simulink model "check_Engine"  (R2018b)
settings: configuration reference "Physics" (kept outside this file)
model workspace (MAT data in the model file):
  veh_param = Simulink.Parameter
  veh_param.Value.cLiftF = 0
  veh_param.Value.cLiftR = 0
  veh_param.Value.CoGx_m = 0
  veh_param.Value.CoGy_m = 0
  veh_param.Value.CoGz_m = 0
  veh_param.Value.cDrag = 0
  veh_param.Value.Aref_m2 = 0
  veh_param.Value.Gearratio = 0
  veh_param.Value.Wheelbase_m = 0
  veh_param.Value.PacLatF = [0 0 0 0 0]
  veh_param.Value.PacLongF = [0 0 0 0 0]
  veh_param.Value.PacLatR = [0 0 0 0 0]
  veh_param.Value.PacLongR = [0 0 0 0 0]
  veh_param.Value.cRollFriction_Npmps = 0
  veh_param.Value.MaxRollFriction_N = 0
  veh_param.Value.T_YawRate_s = 0
  veh_param.Value.T_LatVel_s = 0
  veh_param.Value.TrackWidthF_m = 0
  veh_param.Value.TrackWidthR_m = 0
  veh_param.Value.TireRadiusF_m = 0
  veh_param.Value.TireRadiusR_m = 0
  veh_param.Value.VehicleInertia_kgm2 = 0
  veh_param.Value.WheelInertiaF_kgm2 = 0
  veh_param.Value.WheelInertiaR_kgm2 = 0
  veh_param.Value.VehicleMass_kg = 0
  veh_param.Value.switchModelBlend_mps = 0
  veh_param.Value.PTLimitLowVel_N = 0
  veh_param.Value.switchModelVel_mps = 0
  veh_param.Value.T_Tire_s = 0
  veh_param.DataType = 'struct'
  veh_param.Dimensions = [1 1]
  x0_positionstates = Simulink.Parameter
  x0_positionstates.Value = [0 0 0]
  x0_positionstates.DataType = 'auto'
  x0_positionstates.Dimensions = [1 3]
undefined symbols (not defined in the file): POWTR__DIFFERENTIAL__c_diff_efficiency, POWTR__DIFFERENTIAL__c_diff_ratio, POWTR__DIFFERENTIAL__f_diff_efficiency, POWTR__DIFFERENTIAL__f_diff_ratio, POWTR__DIFFERENTIAL__r_diff_efficiency, POWTR__DIFFERENTIAL__r_diff_ratio, POWTR__ENGINE__n_idle_rpm, POWTR__ENGINE__n_lb_rpm__1, POWTR__ENGINE__n_lb_rpm__2, POWTR__ENGINE__n_lb_rpm__3, POWTR__ENGINE__n_lb_rpm__4, POWTR__ENGINE__n_lb_rpm__5, POWTR__ENGINE__n_lb_rpm__6, POWTR__ENGINE__n_lb_rpm__7, POWTR__ENGINE__n_limit_rpm, POWTR__LAYOUT__p_torque_rear, POWTR__MODE__activate_ThrottleInterface, POWTR__TRANSMISSION__gear__1, POWTR__TRANSMISSION__gear__2, POWTR__TRANSMISSION__gear__3, POWTR__TRANSMISSION__gear__4, POWTR__TRANSMISSION__gear__5, POWTR__TRANSMISSION__gear__6, POWTR__TRANSMISSION__gear__7, POWTR__TRANSMISSION__gear_efficiency__1, POWTR__TRANSMISSION__gear_efficiency__2, POWTR__TRANSMISSION__gear_efficiency__3, POWTR__TRANSMISSION__gear_efficiency__4, POWTR__TRANSMISSION__gear_efficiency__5, POWTR__TRANSMISSION__gear_efficiency__6, POWTR__TRANSMISSION__gear_efficiency__7, POWTR__TRANSMISSION__gear_ratio__1, POWTR__TRANSMISSION__gear_ratio__2, POWTR__TRANSMISSION__gear_ratio__3, POWTR__TRANSMISSION__gear_ratio__4, POWTR__TRANSMISSION__gear_ratio__5, POWTR__TRANSMISSION__gear_ratio__6, POWTR__TRANSMISSION__gear_ratio__7, tireFL__MFSIMPLE__r_tire_m, tireFR__MFSIMPLE__r_tire_m, tireRL__MFSIMPLE__r_tire_m, tireRR__MFSIMPLE__r_tire_m
libraries: simulink x3
settings Model: DataDictionary=vehicleparameters_vehdynsim.sldd  OrderedModelArguments=off  Creator=wischnewski  LastModifiedBy=ga25xiw

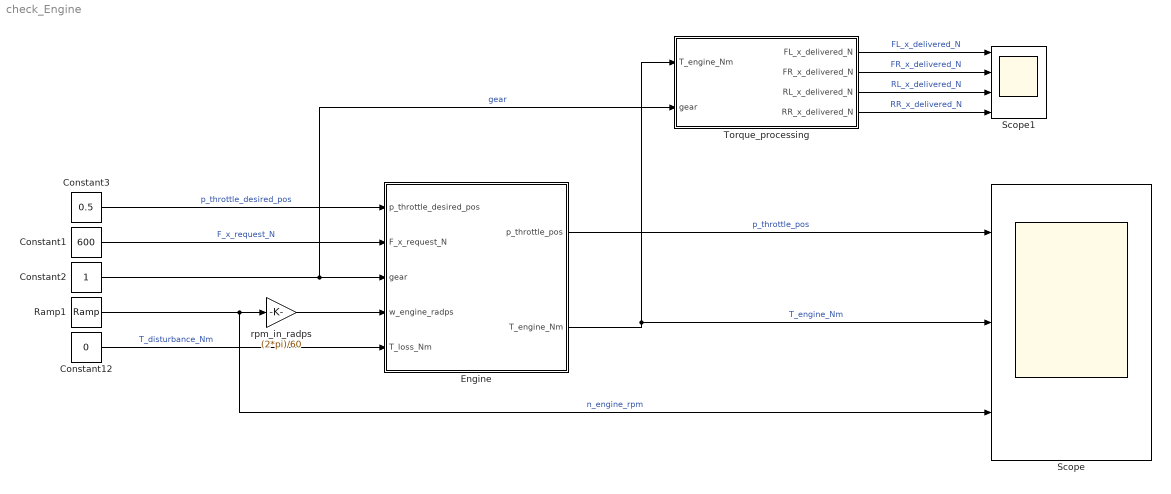
== system check_Engine ==
  Constant1 : Constant  Value=600
  Constant12 : Constant  Value=0
  Constant2 : Constant
  Constant3 : Constant  Value=0.5
  Engine : Subsystem
  Ramp1 : simulink/Sources/Ramp  slope=500  start=0  InitialOutput=2000
  Scope : Scope  NumInputPorts=3
  Scope1 : Scope  NumInputPorts=4
  Torque_processing : Subsystem
  rpm_in_radps : Gain  Gain=(2*pi)/60
  wires:
  Ramp1/1 -> Scope/3, rpm_in_radps/1  "n_engine_rpm"
  Engine/1(p_throttle_pos) -> Scope/1  "p_throttle_pos"
  Torque_processing/1(FL_x_delivered_N) -> Scope1/1  "FL_x_delivered_N"
  Torque_processing/2(FR_x_delivered_N) -> Scope1/2  "FR_x_delivered_N"
  Torque_processing/3(RL_x_delivered_N) -> Scope1/3  "RL_x_delivered_N"
  Torque_processing/4(RR_x_delivered_N) -> Scope1/4  "RR_x_delivered_N"
  Engine/2(T_engine_Nm) -> Torque_processing/1(T_engine_Nm), Scope/2  "T_engine_Nm"
  Constant12/1 -> Engine/5(T_loss_Nm)  "T_disturbance_Nm"
  rpm_in_radps/1 -> Engine/4(w_engine_radps)
  Constant2/1 -> Engine/3(gear), Torque_processing/2(gear)  "gear"
  Constant1/1 -> Engine/2(F_x_request_N)  "F_x_request_N"
  Constant3/1 -> Engine/1(p_throttle_desired_pos)  "p_throttle_desired_pos"

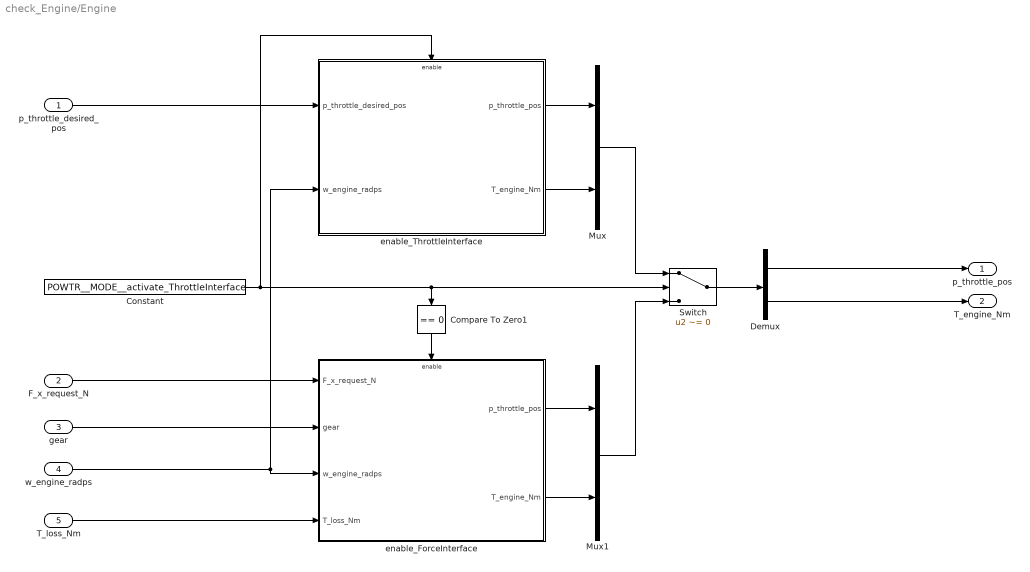
== system check_Engine/Engine ==
  p_throttle_desired_pos : Inport
  F_x_request_N : Inport  Port=2
  gear : Inport  Port=3
  w_engine_radps : Inport  Port=4
  T_loss_Nm : Inport  Port=5
  Compare To Zero1 : simulink/Logic and Bit Operations/Compare To Zero  relop===  OutDataTypeStr=uint8
  Constant : Constant  Value=POWTR__MODE__activate_ThrottleInterface
  Demux : Demux  Outputs=2
  Mux : Mux  Inputs=2
  Mux1 : Mux  Inputs=2
  Switch : Switch  Criteria=u2 ~= 0
  enable_ForceInterface : Subsystem
  enable_ThrottleInterface : Subsystem
  p_throttle_pos : Outport
  T_engine_Nm : Outport  Port=2
  wires:
  Switch/1 -> Demux/1
  Mux1/1 -> Switch/3
  Compare To Zero1/1 -> enable_ForceInterface/Enable
  T_loss_Nm/1 -> enable_ForceInterface/4(T_loss_Nm)
  gear/1 -> enable_ForceInterface/2(gear)
  w_engine_radps/1 -> enable_ForceInterface/3(w_engine_radps), enable_ThrottleInterface/2(w_engine_radps)
  enable_ForceInterface/2(T_engine_Nm) -> Mux1/2
  Constant/1 -> Switch/2, Compare To Zero1/1, enable_ThrottleInterface/Enable
  enable_ForceInterface/1(p_throttle_pos) -> Mux1/1
  F_x_request_N/1 -> enable_ForceInterface/1(F_x_request_N)
  p_throttle_desired_pos/1 -> enable_ThrottleInterface/1(p_throttle_desired_pos)
  enable_ThrottleInterface/2(T_engine_Nm) -> Mux/2
  Mux/1 -> Switch/1
  enable_ThrottleInterface/1(p_throttle_pos) -> Mux/1
  Demux/2 -> T_engine_Nm/1
  Demux/1 -> p_throttle_pos/1

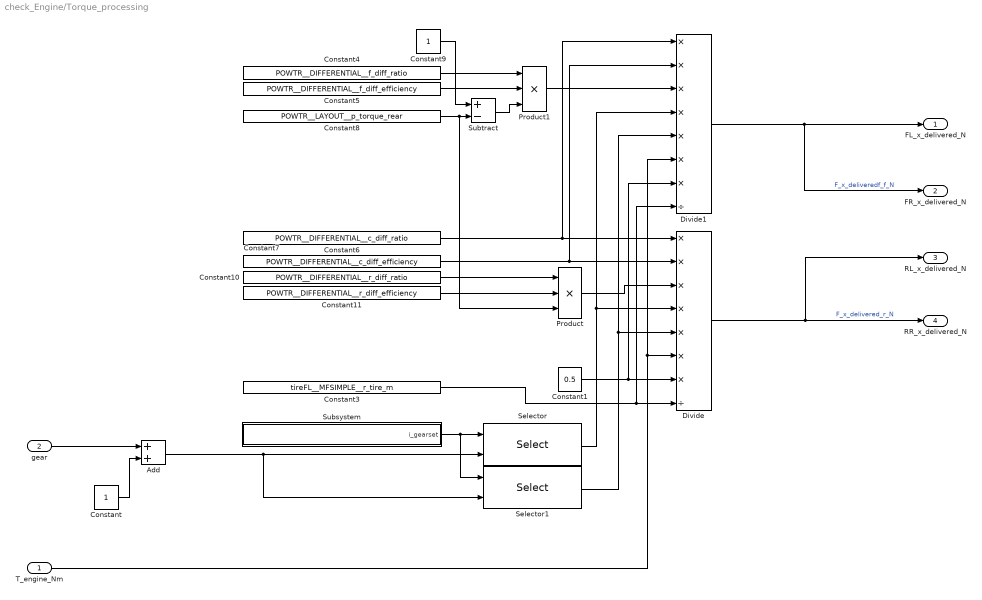
== system check_Engine/Torque_processing ==
  T_engine_Nm : Inport
  gear : Inport  Port=2
  Add : Sum
  Constant : Constant
  Constant1 : Constant  Value=0.5
  Constant10 : Constant  Value=POWTR__DIFFERENTIAL__r_diff_ratio
  Constant11 : Constant  Value=POWTR__DIFFERENTIAL__r_diff_efficiency  VectorParams1D=off
  Constant3 : Constant  Value=tireFL__MFSIMPLE__r_tire_m  VectorParams1D=off
  Constant4 : Constant  Value=POWTR__DIFFERENTIAL__f_diff_ratio
  Constant5 : Constant  Value=POWTR__DIFFERENTIAL__f_diff_efficiency  VectorParams1D=off
  Constant6 : Constant  Value=POWTR__DIFFERENTIAL__c_diff_ratio
  Constant7 : Constant  Value=POWTR__DIFFERENTIAL__c_diff_efficiency
  Constant8 : Constant  Value=POWTR__LAYOUT__p_torque_rear  VectorParams1D=off
  Constant9 : Constant
  Divide : Product  Inputs=*******/
  Divide1 : Product  Inputs=*******/
  Product : Product  Inputs=3
  Product1 : Product  Inputs=3
  Selector : Selector  NumberOfDimensions=2  InputPortWidth=3  IndexOptions=Index vector (dialog),Index vector (port)  Indices=2,1  OutputSizes=1,1
  Selector1 : Selector  NumberOfDimensions=2  InputPortWidth=3  IndexOptions=Index vector (dialog),Index vector (port)  Indices=4,1  OutputSizes=1,1
  Subsystem : Subsystem
  Subtract : Sum  Inputs=+-
  FL_x_delivered_N : Outport
  FR_x_delivered_N : Outport  Port=2
  RL_x_delivered_N : Outport  Port=3
  RR_x_delivered_N : Outport  Port=4
  wires:
  Constant10/1 -> Product/1
  Constant/1 -> Add/2
  Constant8/1 -> Product/3, Subtract/2
  Subsystem/1(i_gearset) -> Selector/1, Selector1/1
  Add/1 -> Selector1/2, Selector/2
  Constant7/1 -> Divide/2, Divide1/2
  Constant9/1 -> Subtract/1
  Constant5/1 -> Product1/2
  Constant6/1 -> Divide/1, Divide1/1
  Subtract/1 -> Product1/3
  Constant4/1 -> Product1/1
  Constant11/1 -> Product/2
  Selector/1 -> Divide/4, Divide1/4
  Selector1/1 -> Divide/5, Divide1/5
  gear/1 -> Add/1
  Product/1 -> Divide/3
  T_engine_Nm/1 -> Divide/6, Divide1/6
  Constant3/1 -> Divide/8, Divide1/8
  Constant1/1 -> Divide/7, Divide1/7
  Product1/1 -> Divide1/3
  Divide/1 -> RL_x_delivered_N/1, RR_x_delivered_N/1  "F_x_delivered_r_N"
  Divide1/1 -> FR_x_delivered_N/1, FL_x_delivered_N/1  "F_x_deliveredf_f_N"

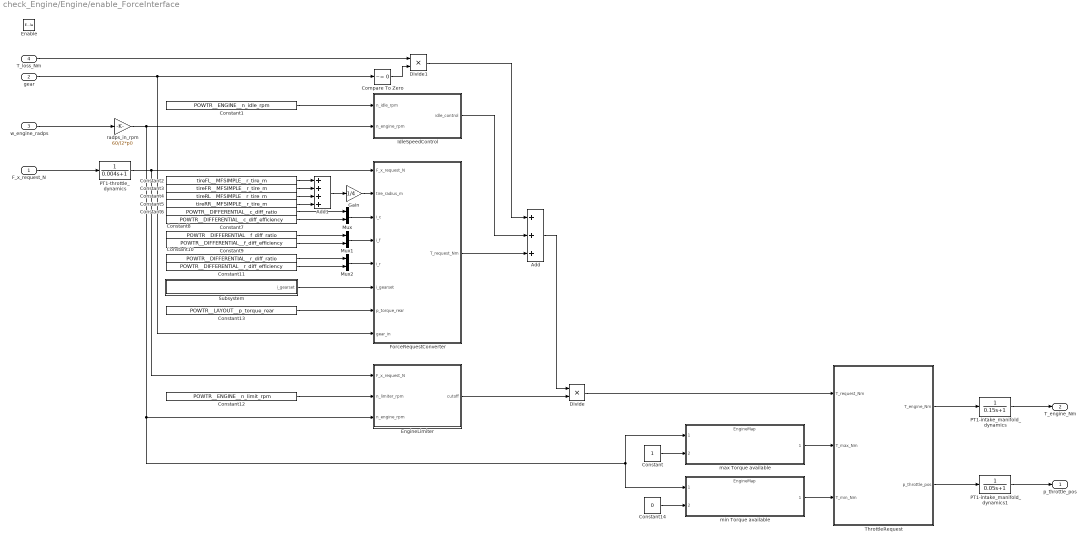
== system check_Engine/Engine/enable_ForceInterface ==
  F_x_request_N : Inport
  gear : Inport  Port=2
  w_engine_radps : Inport  Port=3
  T_loss_Nm : Inport  Port=4
  Enable : EnablePort
  Add : Sum  Inputs=+++
  Add1 : Sum  Inputs=++++
  Compare To Zero : simulink/Logic and Bit Operations/Compare To Zero  relop=~=  OutDataTypeStr=boolean
  Constant : Constant
  Constant1 : Constant  Value=POWTR__ENGINE__n_idle_rpm
  Constant10 : Constant  Value=POWTR__DIFFERENTIAL__r_diff_ratio
  Constant11 : Constant  Value=POWTR__DIFFERENTIAL__r_diff_efficiency
  Constant12 : Constant  Value=POWTR__ENGINE__n_limit_rpm
  Constant13 : Constant  Value=POWTR__LAYOUT__p_torque_rear
  Constant14 : Constant  Value=0
  Constant2 : Constant  Value=tireFL__MFSIMPLE__r_tire_m
  Constant3 : Constant  Value=tireFR__MFSIMPLE__r_tire_m
  Constant4 : Constant  Value=tireRL__MFSIMPLE__r_tire_m
  Constant5 : Constant  Value=tireRR__MFSIMPLE__r_tire_m
  Constant6 : Constant  Value=POWTR__DIFFERENTIAL__c_diff_ratio
  Constant7 : Constant  Value=POWTR__DIFFERENTIAL__c_diff_efficiency
  Constant8 : Constant  Value=POWTR__DIFFERENTIAL__f_diff_ratio
  Constant9 : Constant  Value=POWTR__DIFFERENTIAL__f_diff_efficiency
  Divide : Product  Inputs=**
  Divide1 : Product  Inputs=**
  EngineLimiter : MATLAB Function  TreatAsAtomicUnit=on
  ForceRequestConverter : MATLAB Function  TreatAsAtomicUnit=on
  Gain : Gain  Gain=1/4
  IdleSpeedControl : MATLAB Function  TreatAsAtomicUnit=on
  Mux : Mux  Inputs=2
  Mux1 : Mux  Inputs=2
  Mux2 : Mux  Inputs=2
  PT1-intake_manifold_dynamics : TransferFcn  Denominator=[0.15 1]
  PT1-intake_manifold_dynamics1 : TransferFcn  Denominator=[0.05 1]
  PT1-throttle_dynamics : TransferFcn  Denominator=[0.004 1]
  Subsystem : Subsystem
  ThrottleRequest : MATLAB Function  TreatAsAtomicUnit=on
  max Torque available : ModelReference  ModelNameDialog=EngineMap.slx  SimulationMode=Normal  ModelReferenceVersion=1.393
  min Torque available : ModelReference  ModelNameDialog=EngineMap.slx  SimulationMode=Normal  ModelReferenceVersion=1.393
  radps_in_rpm : Gain  Gain=60/(2*pi)
  p_throttle_pos : Outport
  T_engine_Nm : Outport  Port=2
  wires:
  Constant8/1 -> Mux1/1
  gear/1 -> Compare To Zero/1, ForceRequestConverter/8(gear_in)
  PT1-throttle_dynamics/1 -> ForceRequestConverter/1(F_x_request_N), EngineLimiter/1(F_x_request_N)
  Constant5/1 -> Add1/4
  Constant13/1 -> ForceRequestConverter/7(p_torque_rear)
  Constant7/1 -> Mux/2
  Compare To Zero/1 -> Divide1/2
  T_loss_Nm/1 -> Divide1/1
  EngineLimiter/1(cutoff) -> Divide/2
  Constant3/1 -> Add1/2
  Constant12/1 -> EngineLimiter/2(n_limiter_rpm)
  ForceRequestConverter/1(T_request_Nm) -> Add/3
  Add1/1 -> Gain/1
  IdleSpeedControl/1(idle_control) -> Add/2
  PT1-intake_manifold_dynamics1/1 -> p_throttle_pos/1
  Constant4/1 -> Add1/3
  Mux2/1 -> ForceRequestConverter/5(i_r)
  Divide1/1 -> Add/1
  Constant11/1 -> Mux2/2
  ThrottleRequest/1(T_engine_Nm) -> PT1-intake_manifold_dynamics/1
  Constant10/1 -> Mux2/1
  Mux/1 -> ForceRequestConverter/3(i_c)
  Constant2/1 -> Add1/1
  ThrottleRequest/2(p_throttle_pos) -> PT1-intake_manifold_dynamics1/1
  Mux1/1 -> ForceRequestConverter/4(i_f)
  PT1-intake_manifold_dynamics/1 -> T_engine_Nm/1
  F_x_request_N/1 -> PT1-throttle_dynamics/1
  Add/1 -> Divide/1
  Subsystem/1(i_gearset) -> ForceRequestConverter/6(i_gearset)
  Constant9/1 -> Mux1/2
  w_engine_radps/1 -> radps_in_rpm/1
  Constant1/1 -> IdleSpeedControl/1(n_idle_rpm)
  Gain/1 -> ForceRequestConverter/2(tire_radius_m)
  Constant6/1 -> Mux/1
  Constant14/1 -> min Torque available/2
  radps_in_rpm/1 -> IdleSpeedControl/2(n_engine_rpm), EngineLimiter/3(n_engine_rpm), min Torque available/1, max Torque available/1
  min Torque available/1 -> ThrottleRequest/3(T_min_Nm)
  Divide/1 -> ThrottleRequest/1(T_request_Nm)
  max Torque available/1 -> ThrottleRequest/2(T_max_Nm)
  Constant/1 -> max Torque available/2

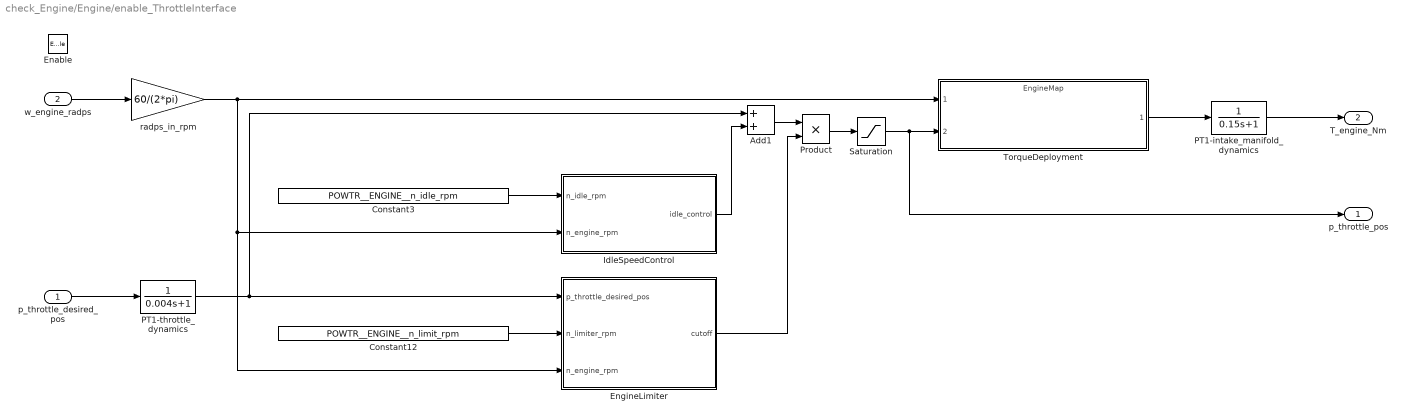
== system check_Engine/Engine/enable_ThrottleInterface ==
  p_throttle_desired_pos : Inport
  w_engine_radps : Inport  Port=2
  Enable : EnablePort
  Add1 : Sum
  Constant12 : Constant  Value=POWTR__ENGINE__n_limit_rpm
  Constant3 : Constant  Value=POWTR__ENGINE__n_idle_rpm
  EngineLimiter : MATLAB Function  TreatAsAtomicUnit=on
  IdleSpeedControl : MATLAB Function  TreatAsAtomicUnit=on
  PT1-intake_manifold_dynamics : TransferFcn  Denominator=[0.15 1]
  PT1-throttle_dynamics : TransferFcn  Denominator=[0.004 1]
  Product : Product
  Saturation : Saturate  UpperLimit=1  LowerLimit=0
  TorqueDeployment : ModelReference  ModelNameDialog=EngineMap.slx  SimulationMode=Normal  ModelReferenceVersion=1.393
  radps_in_rpm : Gain  Gain=60/(2*pi)
  p_throttle_pos : Outport
  T_engine_Nm : Outport  Port=2
  wires:
  Constant12/1 -> EngineLimiter/2(n_limiter_rpm)
  Product/1 -> Saturation/1
  Add1/1 -> Product/1
  EngineLimiter/1(cutoff) -> Product/2
  IdleSpeedControl/1(idle_control) -> Add1/2
  w_engine_radps/1 -> radps_in_rpm/1
  p_throttle_desired_pos/1 -> PT1-throttle_dynamics/1
  Saturation/1 -> TorqueDeployment/2, p_throttle_pos/1
  PT1-intake_manifold_dynamics/1 -> T_engine_Nm/1
  TorqueDeployment/1 -> PT1-intake_manifold_dynamics/1
  radps_in_rpm/1 -> EngineLimiter/3(n_engine_rpm), IdleSpeedControl/2(n_engine_rpm), TorqueDeployment/1
  PT1-throttle_dynamics/1 -> Add1/1, EngineLimiter/1(p_throttle_desired_pos)
  Constant3/1 -> IdleSpeedControl/1(n_idle_rpm)

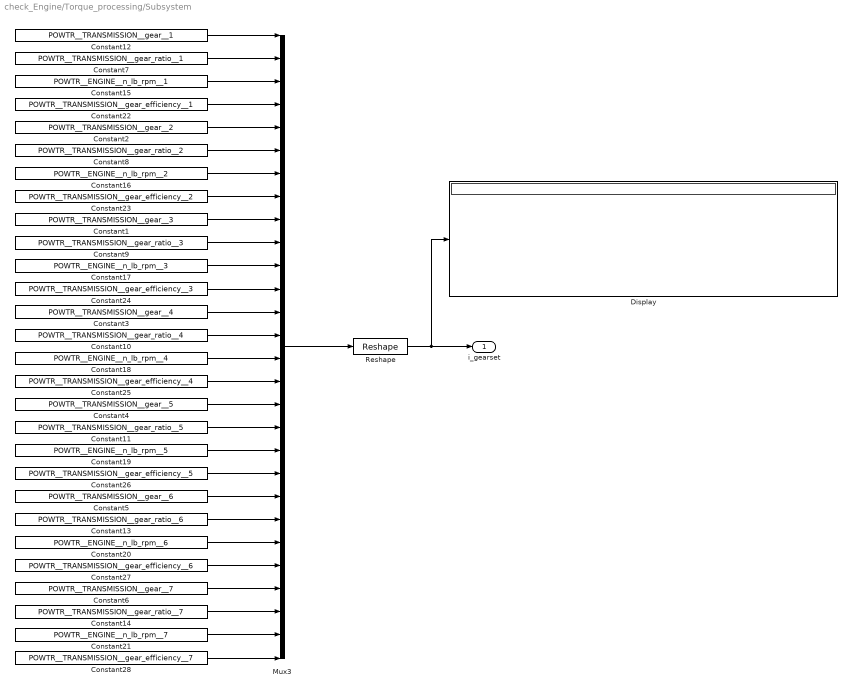
== system check_Engine/Torque_processing/Subsystem ==
  Constant1 : Constant  Value=POWTR__TRANSMISSION__gear__3
  Constant10 : Constant  Value=POWTR__TRANSMISSION__gear_ratio__4
  Constant11 : Constant  Value=POWTR__TRANSMISSION__gear_ratio__5
  Constant12 : Constant  Value=POWTR__TRANSMISSION__gear__1
  Constant13 : Constant  Value=POWTR__TRANSMISSION__gear_ratio__6
  Constant14 : Constant  Value=POWTR__TRANSMISSION__gear_ratio__7
  Constant15 : Constant  Value=POWTR__ENGINE__n_lb_rpm__1
  Constant16 : Constant  Value=POWTR__ENGINE__n_lb_rpm__2
  Constant17 : Constant  Value=POWTR__ENGINE__n_lb_rpm__3
  Constant18 : Constant  Value=POWTR__ENGINE__n_lb_rpm__4
  Constant19 : Constant  Value=POWTR__ENGINE__n_lb_rpm__5
  Constant2 : Constant  Value=POWTR__TRANSMISSION__gear__2
  Constant20 : Constant  Value=POWTR__ENGINE__n_lb_rpm__6
  Constant21 : Constant  Value=POWTR__ENGINE__n_lb_rpm__7
  Constant22 : Constant  Value=POWTR__TRANSMISSION__gear_efficiency__1
  Constant23 : Constant  Value=POWTR__TRANSMISSION__gear_efficiency__2
  Constant24 : Constant  Value=POWTR__TRANSMISSION__gear_efficiency__3
  Constant25 : Constant  Value=POWTR__TRANSMISSION__gear_efficiency__4
  Constant26 : Constant  Value=POWTR__TRANSMISSION__gear_efficiency__5
  Constant27 : Constant  Value=POWTR__TRANSMISSION__gear_efficiency__6
  Constant28 : Constant  Value=POWTR__TRANSMISSION__gear_efficiency__7
  Constant3 : Constant  Value=POWTR__TRANSMISSION__gear__4
  Constant4 : Constant  Value=POWTR__TRANSMISSION__gear__5
  Constant5 : Constant  Value=POWTR__TRANSMISSION__gear__6
  Constant6 : Constant  Value=POWTR__TRANSMISSION__gear__7
  Constant7 : Constant  Value=POWTR__TRANSMISSION__gear_ratio__1
  Constant8 : Constant  Value=POWTR__TRANSMISSION__gear_ratio__2
  Constant9 : Constant  Value=POWTR__TRANSMISSION__gear_ratio__3
  Display : Display
  Mux3 : Mux  Inputs=28
  Reshape : Reshape  OutputDimensionality=Customize  OutputDimensions=[4,7]
  i_gearset : Outport
  wires:
  Mux3/1 -> Reshape/1
  Constant12/1 -> Mux3/1
  Reshape/1 -> i_gearset/1, Display/1
  Constant2/1 -> Mux3/5
  Constant1/1 -> Mux3/9
  Constant3/1 -> Mux3/13
  Constant4/1 -> Mux3/17
  Constant5/1 -> Mux3/21
  Constant6/1 -> Mux3/25
  Constant7/1 -> Mux3/2
  Constant8/1 -> Mux3/6
  Constant9/1 -> Mux3/10
  Constant10/1 -> Mux3/14
  Constant11/1 -> Mux3/18
  Constant13/1 -> Mux3/22
  Constant14/1 -> Mux3/26
  Constant15/1 -> Mux3/3
  Constant16/1 -> Mux3/7
  Constant17/1 -> Mux3/11
  Constant18/1 -> Mux3/15
  Constant19/1 -> Mux3/19
  Constant20/1 -> Mux3/23
  Constant21/1 -> Mux3/27
  Constant22/1 -> Mux3/4
  Constant23/1 -> Mux3/8
  Constant24/1 -> Mux3/12
  Constant25/1 -> Mux3/16
  Constant26/1 -> Mux3/20
  Constant27/1 -> Mux3/24
  Constant28/1 -> Mux3/28

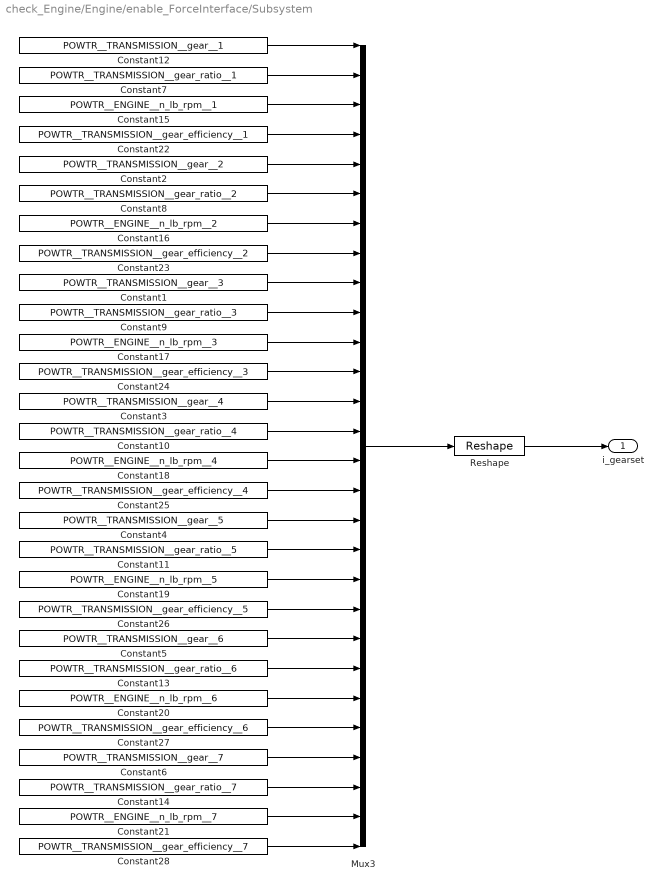
== system check_Engine/Engine/enable_ForceInterface/Subsystem ==
  Constant1 : Constant  Value=POWTR__TRANSMISSION__gear__3
  Constant10 : Constant  Value=POWTR__TRANSMISSION__gear_ratio__4
  Constant11 : Constant  Value=POWTR__TRANSMISSION__gear_ratio__5
  Constant12 : Constant  Value=POWTR__TRANSMISSION__gear__1
  Constant13 : Constant  Value=POWTR__TRANSMISSION__gear_ratio__6
  Constant14 : Constant  Value=POWTR__TRANSMISSION__gear_ratio__7
  Constant15 : Constant  Value=POWTR__ENGINE__n_lb_rpm__1
  Constant16 : Constant  Value=POWTR__ENGINE__n_lb_rpm__2
  Constant17 : Constant  Value=POWTR__ENGINE__n_lb_rpm__3
  Constant18 : Constant  Value=POWTR__ENGINE__n_lb_rpm__4
  Constant19 : Constant  Value=POWTR__ENGINE__n_lb_rpm__5
  Constant2 : Constant  Value=POWTR__TRANSMISSION__gear__2
  Constant20 : Constant  Value=POWTR__ENGINE__n_lb_rpm__6
  Constant21 : Constant  Value=POWTR__ENGINE__n_lb_rpm__7
  Constant22 : Constant  Value=POWTR__TRANSMISSION__gear_efficiency__1
  Constant23 : Constant  Value=POWTR__TRANSMISSION__gear_efficiency__2
  Constant24 : Constant  Value=POWTR__TRANSMISSION__gear_efficiency__3
  Constant25 : Constant  Value=POWTR__TRANSMISSION__gear_efficiency__4
  Constant26 : Constant  Value=POWTR__TRANSMISSION__gear_efficiency__5
  Constant27 : Constant  Value=POWTR__TRANSMISSION__gear_efficiency__6
  Constant28 : Constant  Value=POWTR__TRANSMISSION__gear_efficiency__7
  Constant3 : Constant  Value=POWTR__TRANSMISSION__gear__4
  Constant4 : Constant  Value=POWTR__TRANSMISSION__gear__5
  Constant5 : Constant  Value=POWTR__TRANSMISSION__gear__6
  Constant6 : Constant  Value=POWTR__TRANSMISSION__gear__7
  Constant7 : Constant  Value=POWTR__TRANSMISSION__gear_ratio__1
  Constant8 : Constant  Value=POWTR__TRANSMISSION__gear_ratio__2
  Constant9 : Constant  Value=POWTR__TRANSMISSION__gear_ratio__3
  Mux3 : Mux  Inputs=28
  Reshape : Reshape  OutputDimensionality=Customize  OutputDimensions=[4,7]
  i_gearset : Outport
  wires:
  Mux3/1 -> Reshape/1
  Constant12/1 -> Mux3/1
  Reshape/1 -> i_gearset/1
  Constant2/1 -> Mux3/5
  Constant1/1 -> Mux3/9
  Constant3/1 -> Mux3/13
  Constant4/1 -> Mux3/17
  Constant5/1 -> Mux3/21
  Constant6/1 -> Mux3/25
  Constant7/1 -> Mux3/2
  Constant8/1 -> Mux3/6
  Constant9/1 -> Mux3/10
  Constant10/1 -> Mux3/14
  Constant11/1 -> Mux3/18
  Constant13/1 -> Mux3/22
  Constant14/1 -> Mux3/26
  Constant15/1 -> Mux3/3
  Constant16/1 -> Mux3/7
  Constant17/1 -> Mux3/11
  Constant18/1 -> Mux3/15
  Constant19/1 -> Mux3/19
  Constant20/1 -> Mux3/23
  Constant21/1 -> Mux3/27
  Constant22/1 -> Mux3/4
  Constant23/1 -> Mux3/8
  Constant24/1 -> Mux3/12
  Constant25/1 -> Mux3/16
  Constant26/1 -> Mux3/20
  Constant27/1 -> Mux3/24
  Constant28/1 -> Mux3/28

== matlab function check_Engine/Engine/enable_ThrottleInterface/EngineLimiter ==
  data: p_throttle_desired_pos input; cutoff output; n_limiter_rpm input; n_engine_rpm input
function cutoff = fcn(p_throttle_desired_pos, n_limiter_rpm, n_engine_rpm)

cutoff = EngineLimiter(p_throttle_desired_pos, n_limiter_rpm, n_engine_rpm);

== matlab function check_Engine/Engine/enable_ThrottleInterface/IdleSpeedControl ==
  data: n_idle_rpm input; idle_control output; n_engine_rpm input
function idle_control = fcn(n_idle_rpm, n_engine_rpm)

idle_control = IdleSpeedControl(n_idle_rpm, n_engine_rpm);

== matlab function check_Engine/Engine/enable_ForceInterface/EngineLimiter ==
  data: F_x_request_N input; cutoff output; n_limiter_rpm input; n_engine_rpm input
function cutoff = fcn(F_x_request_N, n_limiter_rpm, n_engine_rpm)

cutoff = EngineLimiter(F_x_request_N, n_limiter_rpm, n_engine_rpm);

== matlab function check_Engine/Engine/enable_ForceInterface/ForceRequestConverter ==
  data: F_x_request_N input; T_request_Nm output; tire_radius_m input; i_c input; i_f input; i_r input; i_gearset input; p_torque_rear input; gear_in input
function T_request_Nm = fcn(F_x_request_N, tire_radius_m, i_c, i_f, i_r, i_gearset, p_torque_rear, gear_in)

T_request_Nm = ForceRequestConverter(F_x_request_N, tire_radius_m, i_c, i_f, i_r, i_gearset, p_torque_rear, gear_in);

== matlab function check_Engine/Engine/enable_ForceInterface/IdleSpeedControl ==
  data: n_idle_rpm input; idle_control output; n_engine_rpm input
function idle_control = fcn(n_idle_rpm, n_engine_rpm)

idle_control = IdleSpeedControl(n_idle_rpm, n_engine_rpm);

== matlab function check_Engine/Engine/enable_ForceInterface/ThrottleRequest ==
  data: T_request_Nm input; T_engine_Nm output; T_max_Nm input; T_min_Nm input; p_throttle_pos output
function [T_engine_Nm, p_throttle_pos] = fcn(T_request_Nm, T_max_Nm, T_min_Nm)

[T_engine_Nm, p_throttle_pos] = ThrottleRequest(T_request_Nm, T_max_Nm, T_min_Nm);
